simulink model "pointmassmodel"  (Simulink 7.9)
settings: Solver=ode3  StartTime=0.0  StopTime=17.0  FixedStep=0.02  RelTol=1e-3
values from neighbouring files (symbols this model uses):
  g = 9.81    [initial.m]    (also in longinvertdynFW.m)
  m = 13.51    [initial.m]    (also in longinvertdynFW.m = 13.5)
  position_0 = [10; 15; -50]    [aerosonde_initialize.m]    (also in initial.m = [0; 5; 50])
  velocity_0 = [23; 0; 0]    [aerosonde_initialize.m]    (also in initial.m = [30; 0; 0])
undefined symbols (not defined in the file or in its folder): pos, root_path
settings Model: Creator=Shihan Tissera  LastModifiedBy=Shihan Tissera

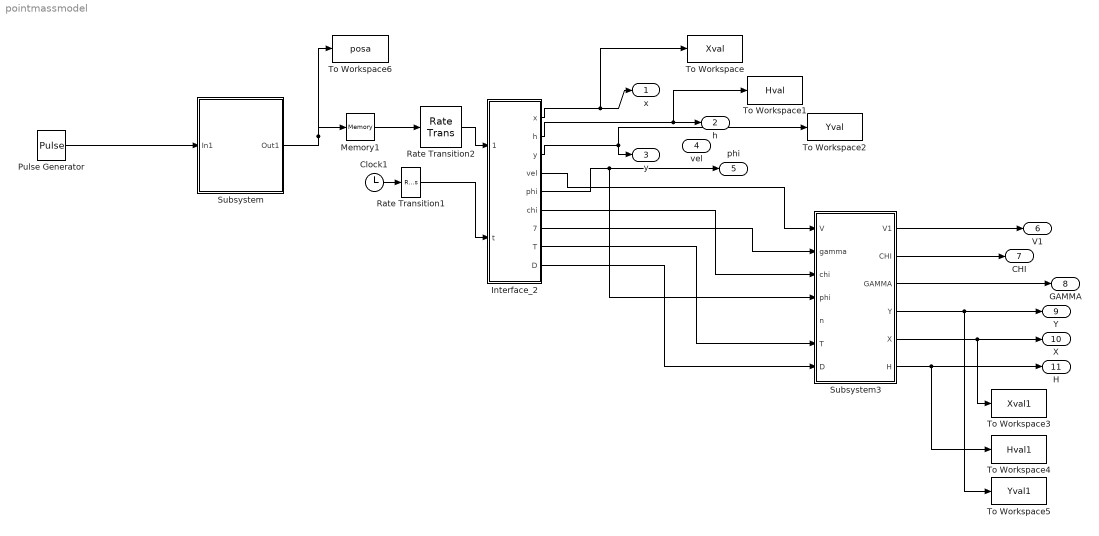
== system pointmassmodel ==
  Clock1 : Clock
  Interface_2 : MATLAB Function  TreatAsAtomicUnit=on
  Memory1 : Memory  X0=pos
  Pulse Generator : DiscretePulseGenerator  PulseType=Time based  Period=22  PulseWidth=2/22
  Rate Transition1 : RateTransition
  Rate Transition2 : RateTransition  X0=pos
  Subsystem : Subsystem
  Subsystem3 : Subsystem
  To Workspace : ToWorkspace  VariableName=Xval  SampleTime=-1
  To Workspace1 : ToWorkspace  VariableName=Hval  SampleTime=-1
  To Workspace2 : ToWorkspace  VariableName=Yval  SampleTime=-1
  To Workspace3 : ToWorkspace  VariableName=Xval1  SampleTime=-1
  To Workspace4 : ToWorkspace  VariableName=Hval1  SampleTime=-1
  To Workspace5 : ToWorkspace  VariableName=Yval1  SampleTime=-1
  To Workspace6 : ToWorkspace  VariableName=posa  SampleTime=-1
  x : Outport
  h : Outport  Port=2
  y : Outport  Port=3
  vel : Outport  Port=4
  phi : Outport  Port=5
  V1 : Outport  Port=6
  CHI : Outport  Port=7
  GAMMA : Outport  Port=8
  Y : Outport  Port=9
  X : Outport  Port=10
  H : Outport  Port=11
  wires:
  Clock1/1 -> Rate Transition1/1
  Interface_2/1(x) -> x/1, To Workspace/1
  Interface_2/2(h) -> h/1, To Workspace1/1
  Interface_2/3(y) -> y/1, To Workspace2/1
  Interface_2/5(phi) -> phi/1, Subsystem3/4(phi)
  Rate Transition2/1 -> Interface_2/1(Input)
  Rate Transition1/1 -> Interface_2/2(t)
  Memory1/1 -> Rate Transition2/1
  Pulse Generator/1 -> Subsystem/1(In1)
  Subsystem/1(Out1) -> Memory1/1, To Workspace6/1
  Subsystem3/1(V1) -> V1/1
  Subsystem3/2(CHI) -> CHI/1
  Subsystem3/3(GAMMA) -> GAMMA/1
  Subsystem3/4(Y) -> Y/1, To Workspace5/1
  Subsystem3/5(X) -> X/1, To Workspace3/1
  Subsystem3/6(H) -> H/1, To Workspace4/1
  Interface_2/7(gamma) -> Subsystem3/2(gamma)
  Interface_2/6(chi) -> Subsystem3/3(chi)
  Interface_2/4(vel) -> Subsystem3/1(V)
  ? -> Subsystem3/5(n)
  Interface_2/8(T) -> Subsystem3/6(T)
  Interface_2/9(D) -> Subsystem3/7(D)

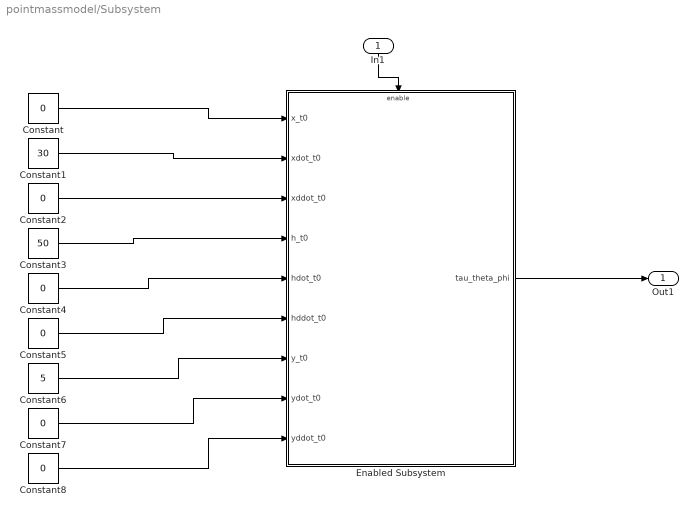
== system pointmassmodel/Subsystem ==
  In1 : Inport
  Constant{,2,4..5,7..8} (6 alike) : Constant  Value=0
  Constant1 : Constant  Value=30
  Constant3 : Constant  Value=50
  Constant6 : Constant  Value=5
  Enabled Subsystem : Subsystem  TreatAsAtomicUnit=on
  Out1 : Outport
  wires:
  In1/1 -> Enabled Subsystem/Enable
  Enabled Subsystem/1(tau_theta_phi) -> Out1/1
  Constant/1 -> Enabled Subsystem/1(x_t0)
  Constant1/1 -> Enabled Subsystem/2(xdot_t0)
  Constant2/1 -> Enabled Subsystem/3(xddot_t0)
  Constant3/1 -> Enabled Subsystem/4(h_t0)
  Constant4/1 -> Enabled Subsystem/5(hdot_t0)
  Constant5/1 -> Enabled Subsystem/6(hddot_t0)
  Constant6/1 -> Enabled Subsystem/7(y_t0)
  Constant7/1 -> Enabled Subsystem/8(ydot_t0)
  Constant8/1 -> Enabled Subsystem/9(yddot_t0)

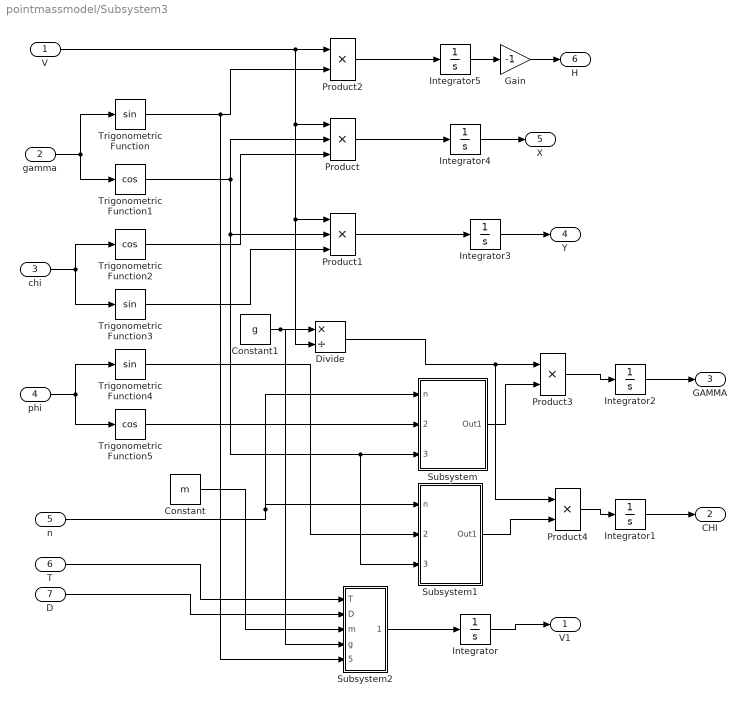
== system pointmassmodel/Subsystem3 ==
  V : Inport
  gamma : Inport  Port=2
  chi : Inport  Port=3
  phi : Inport  Port=4
  n : Inport  Port=5
  T : Inport  Port=6
  D : Inport  Port=7
  Constant : Constant  Value=m
  Constant1 : Constant  Value=g
  Divide : Product  Inputs=*/
  Gain : Gain  Gain=-1
  Integrator{,1..2,4} (4 alike) : Integrator
  Integrator3 : Integrator  InitialCondition=5
  Integrator5 : Integrator  InitialCondition=-50
  Product : Product  Inputs=3  RndMeth=Zero
  Product1 : Product  Inputs=3  RndMeth=Zero
  Product2 : Product  RndMeth=Zero
  Product3 : Product  RndMeth=Zero
  Product4 : Product  RndMeth=Zero
  Subsystem : Subsystem
  Subsystem1 : Subsystem
  Subsystem2 : Subsystem
  Trigonometric Function : Trigonometry
  Trigonometric Function1 : Trigonometry  Operator=cos
  Trigonometric Function2 : Trigonometry  Operator=cos
  Trigonometric Function3 : Trigonometry
  Trigonometric Function4 : Trigonometry
  Trigonometric Function5 : Trigonometry  Operator=cos
  V1 : Outport
  CHI : Outport  Port=2
  GAMMA : Outport  Port=3
  Y : Outport  Port=4
  X : Outport  Port=5
  H : Outport  Port=6
  wires:
  gamma/1 -> Trigonometric Function/1, Trigonometric Function1/1
  chi/1 -> Trigonometric Function2/1, Trigonometric Function3/1
  phi/1 -> Trigonometric Function4/1, Trigonometric Function5/1
  Trigonometric Function1/1 -> Product/2, Product1/2, Subsystem/3(cos(gamma)), Subsystem1/3(cos(gamma))
  Trigonometric Function2/1 -> Product/3
  Trigonometric Function3/1 -> Product1/3
  Trigonometric Function/1 -> Product2/2, Subsystem2/5(sin(gamma))
  V/1 -> Product2/1, Product/1, Product1/1, Divide/2
  Subsystem/1(Out1) -> Product3/2
  Divide/1 -> Product3/1, Product4/1
  n/1 -> Subsystem/1(n), Subsystem1/1(n)
  Trigonometric Function5/1 -> Subsystem/2(cos(phi))
  Trigonometric Function4/1 -> Subsystem1/2(sin(phi))
  Subsystem1/1(Out1) -> Product4/2
  T/1 -> Subsystem2/1(T)
  D/1 -> Subsystem2/2(D)
  Constant/1 -> Subsystem2/3(m)
  Constant1/1 -> Divide/1, Subsystem2/4(g)
  Subsystem2/1(Out1) -> Integrator/1
  Integrator/1 -> V1/1
  Product4/1 -> Integrator1/1
  Integrator1/1 -> CHI/1
  Product3/1 -> Integrator2/1
  Integrator2/1 -> GAMMA/1
  Integrator3/1 -> Y/1
  Product1/1 -> Integrator3/1
  Integrator4/1 -> X/1
  Product/1 -> Integrator4/1
  Product2/1 -> Integrator5/1
  Integrator5/1 -> Gain/1
  Gain/1 -> H/1

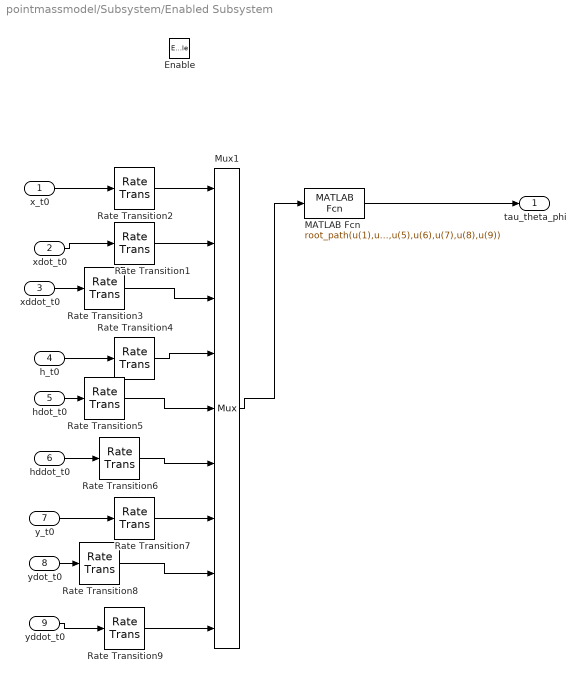
== system pointmassmodel/Subsystem/Enabled Subsystem ==
  x_t0 : Inport
  xdot_t0 : Inport  Port=2
  xddot_t0 : Inport  Port=3
  h_t0 : Inport  Port=4
  hdot_t0 : Inport  Port=5
  hddot_t0 : Inport  Port=6
  y_t0 : Inport  Port=7
  ydot_t0 : Inport  Port=8
  yddot_t0 : Inport  Port=9
  Enable : EnablePort  StatesWhenEnabling=reset
  MATLAB Fcn : MATLABFcn  MATLABFcn=root_path(u(1),u(2),u(3),u(4),u(5),u(6),u(7),u(8),u(9))  OutputDimensions=[850 9]  Output1D=off
  Mux1 : Mux  Inputs=9
  Rate Transition1 : RateTransition  X0=velocity_0(1)
  Rate Transition2 : RateTransition  X0=position_0(1)
  Rate Transition3 : RateTransition
  Rate Transition4 : RateTransition  X0=position_0(3)
  Rate Transition5 : RateTransition  X0=velocity_0(3)
  Rate Transition6 : RateTransition
  Rate Transition7 : RateTransition  X0=position_0(2)
  Rate Transition8 : RateTransition  X0=velocity_0(2)
  Rate Transition9 : RateTransition
  tau_theta_phi : Outport
  wires:
  x_t0/1 -> Rate Transition2/1
  xdot_t0/1 -> Rate Transition1/1
  xddot_t0/1 -> Rate Transition3/1
  h_t0/1 -> Rate Transition4/1
  hdot_t0/1 -> Rate Transition5/1
  hddot_t0/1 -> Rate Transition6/1
  y_t0/1 -> Rate Transition7/1
  ydot_t0/1 -> Rate Transition8/1
  yddot_t0/1 -> Rate Transition9/1
  MATLAB Fcn/1 -> tau_theta_phi/1
  Mux1/1 -> MATLAB Fcn/1
  Rate Transition2/1 -> Mux1/1
  Rate Transition1/1 -> Mux1/2
  Rate Transition3/1 -> Mux1/3
  Rate Transition4/1 -> Mux1/4
  Rate Transition5/1 -> Mux1/5
  Rate Transition6/1 -> Mux1/6
  Rate Transition7/1 -> Mux1/7
  Rate Transition8/1 -> Mux1/8
  Rate Transition9/1 -> Mux1/9

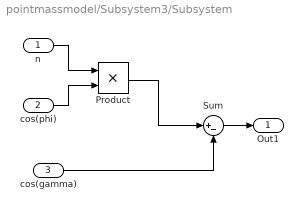
== system pointmassmodel/Subsystem3/Subsystem ==
  n : Inport
  cos(phi) : Inport  Port=2
  cos(gamma) : Inport  Port=3
  Product : Product  RndMeth=Zero
  Sum : Sum  Inputs=|+-
  Out1 : Outport
  wires:
  n/1 -> Product/1
  cos(phi)/1 -> Product/2
  Product/1 -> Sum/1
  cos(gamma)/1 -> Sum/2
  Sum/1 -> Out1/1

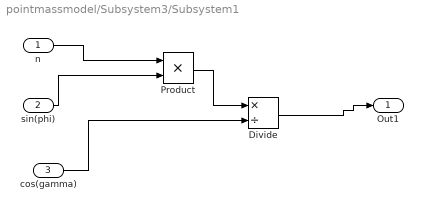
== system pointmassmodel/Subsystem3/Subsystem1 ==
  n : Inport
  sin(phi) : Inport  Port=2
  cos(gamma) : Inport  Port=3
  Divide : Product  Inputs=*/
  Product : Product  RndMeth=Zero
  Out1 : Outport
  wires:
  n/1 -> Product/1
  sin(phi)/1 -> Product/2
  Divide/1 -> Out1/1
  cos(gamma)/1 -> Divide/2
  Product/1 -> Divide/1

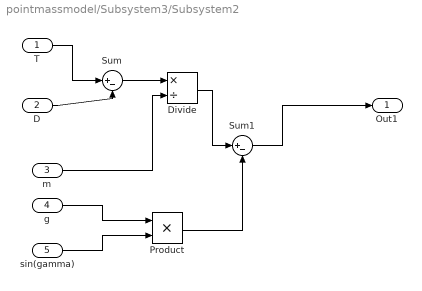
== system pointmassmodel/Subsystem3/Subsystem2 ==
  T : Inport
  D : Inport  Port=2
  m : Inport  Port=3
  g : Inport  Port=4
  sin(gamma) : Inport  Port=5
  Divide : Product  Inputs=*/
  Product : Product  RndMeth=Zero
  Sum : Sum  Inputs=|+-
  Sum1 : Sum  Inputs=|+-
  Out1 : Outport
  wires:
  Sum1/1 -> Out1/1
  T/1 -> Sum/1
  D/1 -> Sum/2
  Sum/1 -> Divide/1
  m/1 -> Divide/2
  Divide/1 -> Sum1/1
  g/1 -> Product/1
  sin(gamma)/1 -> Product/2
  Product/1 -> Sum1/2

== matlab function Interface_2 ==
  data: Input input double; t input double; x output double; h output double; y output double; vel output double; phi output double; chi output double; gamma output double; T output double; D output double
function [x,h,y,vel,phi,chi,gamma,T,D]  = fcn(Input,t)
% % %#codegen
% j=1+10*t;
% j=floor(j);
% if j>10
%     j=mod(j,10);
% % j=j-10;
% end
ts=0.02;
m=mod(floor(1/ts*t),849);
j=m+1;
if m==0
    if t>0
    j=850;
    end
end
% P=Input(j,1:3);
% dP=Input(j,4:6);
% d2P=Input(j,7:9);
% d3P=Input(j,10:12);
% out=TrP=Input(j,1:3);
x=Input(j,1);
h=Input(j,2);
y=Input(j,3);
vel=Input(j,4);
phi=Input(j,5);
chi=Input(j,6);
gamma=Input(j,7);
T=Input(j,8);
D=Input(j,9);
